simulink model "SSModel_USUnits"  (R2020b)
settings: Solver=FixedStepAuto  StartTime=0.0  StopTime=100  FixedStep=0.02  RelTol=1e-3
libraries: Lib_Solve_SSNRSolverJC_EMTAT x2, PB_Library_Master x1
settings Model: Creator=gfretti  LastModifiedBy=nbutler2
settings SFSimCC: CustomCodeUndefinedFunction=UseInterfaceOnly

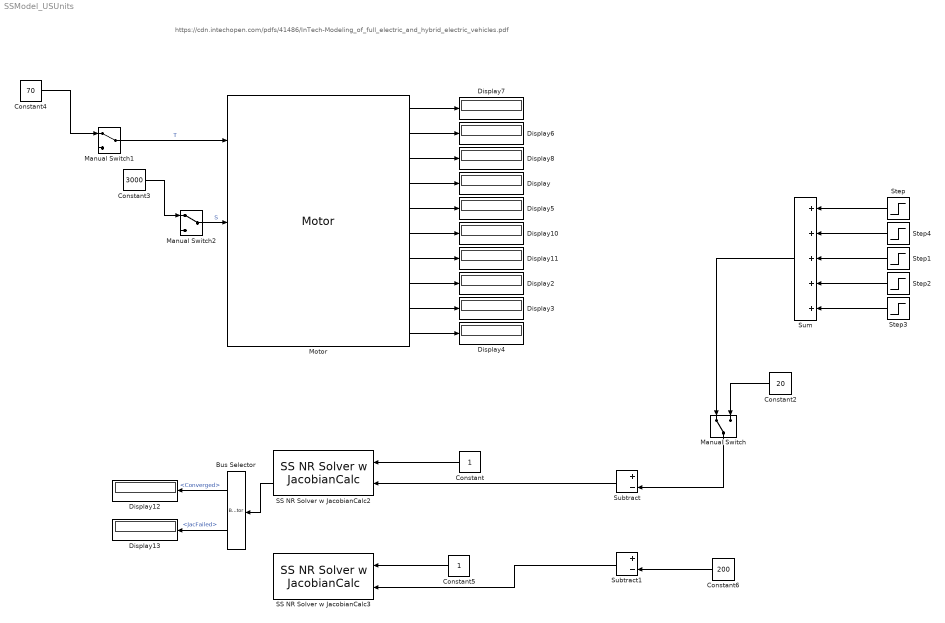
== system SSModel_USUnits ==
  note: https://cdn.intechopen.com/pdfs/41486/InTech-Modeling_of_full_electric_and_hybrid_electric_vehicles.pdf
  Bus Selector : BusSelector  OutputSignals=Converged,JacFailed
  Constant : Constant
  Constant2 : Constant  Value=20
  Constant3 : Constant  Value=3000
  Constant4 : Constant  Value=70
  Constant5 : Constant
  Constant6 : Constant  Value=200
  Display{,2..8,10..13} (12 alike) : Display
  Manual Switch : ManualSwitch
  Manual Switch1 : ManualSwitch
  Manual Switch2 : ManualSwitch
  Motor : PB_Library_Master/Motor  pp=2.5  flux_m=0.46219  R_s=0.032  L_s=0.00115  P_Fe_Nom=904.3614  S_nom=3000  T_nom=70  P_out_max=22000  I_max=36.5  P_in_max=30000  T_max=80  MassEst_M=136.5892  Poles_i=5  R_s_i=.032  L_s_i=.00086+0.00029  S_nom_i=3000  T_nom_i=70  P_out_max_i=22000  I_max_i=36.5  P_in_max_i=30000  K_i=121  V_nom_i=368  T_max_i=80  CalculatePFe=Compute iron losses automatically  P_Fe_Nom_i=0  I_nom_i=36.5  PF_nom_i=0.99  P_Fe_Calc_Flag=1
  SS NR Solver w JacobianCalc2 : Lib_Solve_SSNRSolverJC_EMTAT/SS NR Solver w JacobianCalc  SJac_Per_M=[-0.01;0.01]  SNR_IC_M=10  SNR_DX_M=100  SNR_Mx_M=100000  SNR_Mn_M=0.00001  SJacobianAttempts_M=20000  Cond_Limits_M=0.01
  SS NR Solver w JacobianCalc3 : Lib_Solve_SSNRSolverJC_EMTAT/SS NR Solver w JacobianCalc  SJac_Per_M=[-0.01;0.01]  SNR_IC_M=150  SNR_DX_M=100  SNR_Mx_M=100000  SNR_Mn_M=0.00001  SJacobianAttempts_M=20000  Cond_Limits_M=0.01
  Step : Step  Time=10  After=5  SampleTime=0
  Step1 : Step  Time=30  After=5  SampleTime=0
  Step2 : Step  Time=40  After=-5  SampleTime=0
  Step3 : Step  Time=50  After=-5  SampleTime=0
  Step4 : Step  Time=20  After=5  SampleTime=0
  Subtract : Sum  Inputs=+-
  Subtract1 : Sum  Inputs=+-
  Sum : Sum  Inputs=+++++
  wires:
  Motor/4 -> Display/1
  Motor/8 -> Display2/1
  Motor/9 -> Display3/1
  Motor/10 -> Display4/1
  Motor/5 -> Display5/1
  Motor/1 -> Display7/1
  Motor/3 -> Display8/1
  Motor/6 -> Display10/1
  Motor/7 -> Display11/1
  Constant/1 -> SS NR Solver w JacobianCalc2/1
  Motor/2 -> Display6/1
  Subtract/1 -> SS NR Solver w JacobianCalc2/2
  Manual Switch/1 -> Subtract/2
  Constant2/1 -> Manual Switch/2
  SS NR Solver w JacobianCalc2/2 -> Bus Selector/1
  Bus Selector/2 -> Display13/1  "<JacFailed>"
  Bus Selector/1 -> Display12/1  "<Converged>"
  Step/1 -> Sum/1
  Sum/1 -> Manual Switch/1
  Step4/1 -> Sum/2
  Step1/1 -> Sum/3
  Step2/1 -> Sum/4
  Step3/1 -> Sum/5
  Manual Switch1/1 -> Motor/1  "T"
  Constant4/1 -> Manual Switch1/1
  Manual Switch2/1 -> Motor/2  "S"
  Constant3/1 -> Manual Switch2/1
  Constant5/1 -> SS NR Solver w JacobianCalc3/1
  Subtract1/1 -> SS NR Solver w JacobianCalc3/2
  Constant6/1 -> Subtract1/2
